simulink model "thermostat"  (R2025b)
settings: Solver=VariableStepAuto  StartTime=0.0  StopTime=10.0  RelTol=1e-3
libraries: simulink x1
settings Model: Creator=hahnc  LastModifiedBy=hahnc

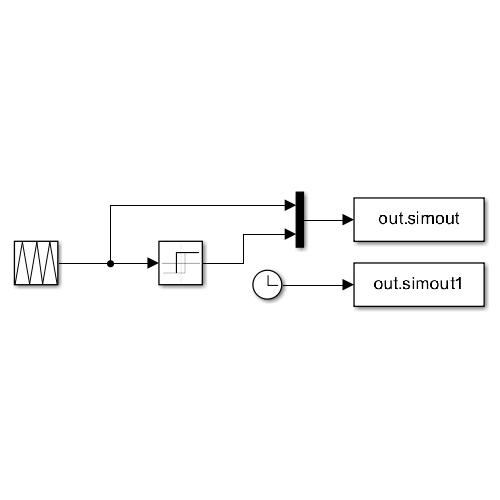
[thumbnail: Simulink's stored preview of the top-level diagram]
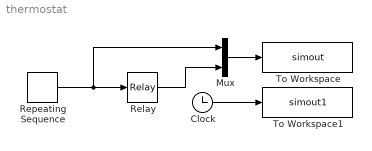
== system thermostat ==
  Clock : Clock
  Mux : Mux  Inputs=2
  Relay : Relay  OnSwitchValue=5*(5/9)  OffSwitchValue=-5*(5/9)
  Repeating Sequence : simulink/Sources/Repeating Sequence  rep_seq_t=[0 3 6]  rep_seq_y=[-4 4 -4]
  To Workspace : ToWorkspace  VariableName=simout  SampleTime=-1
  To Workspace1 : ToWorkspace  VariableName=simout1  SampleTime=-1
  wires:
  Repeating Sequence/1 -> Mux/1, Relay/1
  Mux/1 -> To Workspace/1
  Relay/1 -> Mux/2
  Clock/1 -> To Workspace1/1
